simulink model "GlideslopeAndFlare"  (R2021b)
settings: Solver=VariableStepAuto  StartTime=0.0  StopTime=150  RelTol=1e-3
values from neighbouring files (symbols this model uses):
  alpha0 = trim_state_lo(8)    [Glideslope.m]
  coeff_x = x0/sqrt(x0^2+y0^2)    [Glideslope.m]
  coeff_y = y0/sqrt(x0^2+y0^2)    [Glideslope.m]
  h_flare = 19.1817    [Glideslope.m]
  max_dev_elevator = 25 - trim_control_lo(1)    [Glideslope.m]
  max_dev_thrust = 19000 - trim_thrust_lo    [Glideslope.m]
  min_dev_elevator = -25 - trim_control_lo(1)    [Glideslope.m]
  min_dev_thrust = 1000 - trim_thrust_lo    [Glideslope.m]
  tau = 1.2217    [Glideslope.m]
  theta0 = trim_state_lo(5)    [Glideslope.m]
  x0 = 3000 + 2000/(3*pi/180)    (= 41197.1863421)    [Glideslope.m]
undefined symbols (not defined in the file or in its folder): magnitude
libraries: slpidlib x2, cstblocks x1
settings Model: Creator=misha  LastModifiedBy=20181021

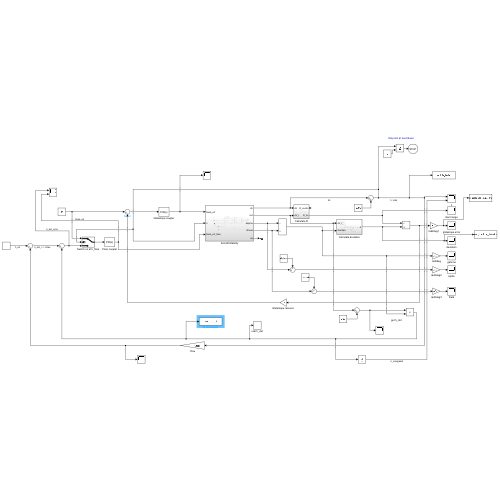
[thumbnail: Simulink's stored preview of the top-level diagram]
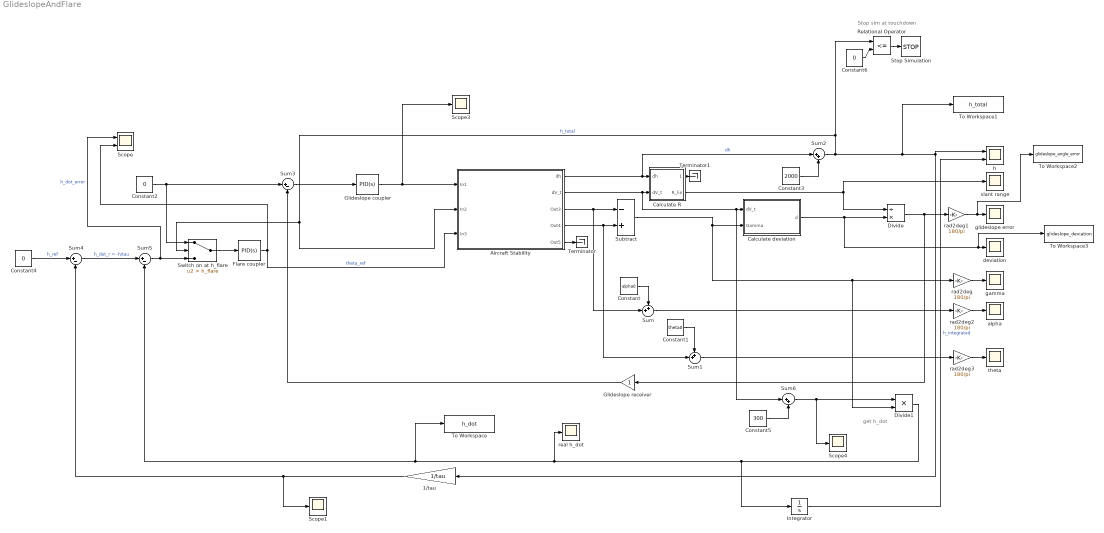
== system GlideslopeAndFlare ==
  note: Stop sim at touchdown
  note: get h_dot
  1/tau : Gain  Gain=1/tau
  Aircraft Stability : Subsystem
  Calculate R : Subsystem
  Calculate deviation : Subsystem
  Constant : Constant  Value=alpha0
  Constant1 : Constant  Value=theta0
  Constant2 : Constant  Value=0
  Constant3 : Constant  Value=2000
  Constant4 : Constant  Value=0
  Constant5 : Constant  Value=300
  Constant6 : Constant  Value=0
  Divide : Product  Inputs=/*
  Divide1 : Product  Inputs=**
  Flare coupler : slpidlib/PID Controller  Controller=PID  Form=Parallel  TimeDomain=Continuous-time  UseExternalTs=off  SampleTime=-1  IntegratorMethod=Forward Euler  FilterMethod=Forward Euler  ControllerParametersSource=internal  P=0.205  I=0.0205  D=0  UseFilter=on  N=100  TunerSelectOption=Transfer Function Based (PID Tuner App)  InitialConditionSource=internal  InitialConditionForIntegrator=0  InitialConditionForFilter=0  DifferentiatorICPrevScaledInput=0  ExternalReset=none  TrackingMode=off  Kt=1  LimitOutput=off  SatLimitsSource=internal  UpperSaturationLimit=inf  LowerSaturationLimit=-inf  LinearizeAsGain=on  AntiWindupMode=none  Kb=1  POutMin=[]  POutMax=[]  IOutMin=[]  IOutMax=[]  DOutMin=[]  DOutMax=[]  NOutMin=[]  NOutMax=[]  SumOutMin=[]  SumOutMax=[]  SaturationOutMin=[]  SaturationOutMax=[]  PParamMin=[]  PParamMax=[]  IParamMin=[]  IParamMax=[]  DParamMin=[]  DParamMax=[]  NParamMin=[]  NParamMax=[]  KbParamMin=[]  KbParamMax=[]  KtParamMin=[]  KtParamMax=[]  KbOutMin=[]  KbOutMax=[]  KtOutMin=[]  KtOutMax=[]  IntegratorOutMin=[]  IntegratorOutMax=[]  FilterOutMin=[]  FilterOutMax=[]  SumI1OutMin=[]  SumI1OutMax=[]  SumI2OutMin=[]  SumI2OutMax=[]  SumI3OutMin=[]  SumI3OutMax=[]  SumI4OutMin=[]  SumI4OutMax=[]  SumDOutMin=[]  SumDOutMax=[]  DifferentiatorOutMin=[]  DifferentiatorOutMax=[]  FilterDiffOutCoefMin=[]  FilterDiffOutCoefMax=[]  ReciprocalOutMin=[]  ReciprocalOutMax=[]  SumDenOutMin=[]  SumDenOutMax=[]  SumNumOutMin=[]  SumNumOutMax=[]  DivideOutMin=[]  DivideOutMax=[]  UdiffTsProdOutMin=[]  UdiffTsProdOutMax=[]  NTsProdOutMin=[]  NTsProdOutMax=[]  UintegralTsProdOutMin=[]  UintegralTsProdOutMax=[]  UngainTsProdOutMin=[]  UngainTsProdOutMax=[]  IntegratorContinuousStateAttributes=''  IntegratorStateMustResolveToSignalObject=off  IntegratorRTWStateStorageClass=Auto  FilterContinuousStateAttributes=''  FilterStateMustResolveToSignalObject=off  FilterRTWStateStorageClass=Auto  ParallelPVariant=InternalParameters  IdealPVariant=Disabled  IVariant=InternalParameters  DVariant=InternalParameters  IntegratorVariant=Continuous  SatVariant=Disabled  AWVariant=Passthrough  PCopyVariant=Disabled  TRVariant=Disabled  FdbkBlocksVariant=Forward  IdealPFdbkVariant=Disabled  SatFdbkVariant=Disabled  DerivativeFilterVariant=ContFilter  NVariant=InternalParameters  NCopyVariant=Disabled  FilterICVariant=InternalICsFilter  IntegratorICVariant=InternalICs  ExternalResetVariant=Disabled  TRSumVariant=Passthrough  SumFdbkVariant=Disabled  SumVariant=Sum_PID  TsampFilterVariant=InternalTs  TsampNgainVariant=Passthrough  TsampIntegralVariant=Passthrough  ExternalSaturationOutDataTypeStr=Inherit: Same as second input
  Glideslope coupler : slpidlib/PID Controller  Controller=PID  Form=Parallel  TimeDomain=Continuous-time  UseExternalTs=off  SampleTime=-1  IntegratorMethod=Forward Euler  FilterMethod=Forward Euler  ControllerParametersSource=internal  P=2000  I=200  D=0  UseFilter=on  N=100  TunerSelectOption=Transfer Function Based (PID Tuner App)  InitialConditionSource=internal  InitialConditionForIntegrator=0  InitialConditionForFilter=0  DifferentiatorICPrevScaledInput=0  ExternalReset=none  TrackingMode=off  Kt=1  LimitOutput=off  SatLimitsSource=internal  UpperSaturationLimit=inf  LowerSaturationLimit=-inf  LinearizeAsGain=on  AntiWindupMode=none  Kb=1  POutMin=[]  POutMax=[]  IOutMin=[]  IOutMax=[]  DOutMin=[]  DOutMax=[]  NOutMin=[]  NOutMax=[]  SumOutMin=[]  SumOutMax=[]  SaturationOutMin=[]  SaturationOutMax=[]  PParamMin=[]  PParamMax=[]  IParamMin=[]  IParamMax=[]  DParamMin=[]  DParamMax=[]  NParamMin=[]  NParamMax=[]  KbParamMin=[]  KbParamMax=[]  KtParamMin=[]  KtParamMax=[]  KbOutMin=[]  KbOutMax=[]  KtOutMin=[]  KtOutMax=[]  IntegratorOutMin=[]  IntegratorOutMax=[]  FilterOutMin=[]  FilterOutMax=[]  SumI1OutMin=[]  SumI1OutMax=[]  SumI2OutMin=[]  SumI2OutMax=[]  SumI3OutMin=[]  SumI3OutMax=[]  SumI4OutMin=[]  SumI4OutMax=[]  SumDOutMin=[]  SumDOutMax=[]  DifferentiatorOutMin=[]  DifferentiatorOutMax=[]  FilterDiffOutCoefMin=[]  FilterDiffOutCoefMax=[]  ReciprocalOutMin=[]  ReciprocalOutMax=[]  SumDenOutMin=[]  SumDenOutMax=[]  SumNumOutMin=[]  SumNumOutMax=[]  DivideOutMin=[]  DivideOutMax=[]  UdiffTsProdOutMin=[]  UdiffTsProdOutMax=[]  NTsProdOutMin=[]  NTsProdOutMax=[]  UintegralTsProdOutMin=[]  UintegralTsProdOutMax=[]  UngainTsProdOutMin=[]  UngainTsProdOutMax=[]  IntegratorContinuousStateAttributes=''  IntegratorStateMustResolveToSignalObject=off  IntegratorRTWStateStorageClass=Auto  FilterContinuousStateAttributes=''  FilterStateMustResolveToSignalObject=off  FilterRTWStateStorageClass=Auto  ParallelPVariant=InternalParameters  IdealPVariant=Disabled  IVariant=InternalParameters  DVariant=InternalParameters  IntegratorVariant=Continuous  SatVariant=Disabled  AWVariant=Passthrough  PCopyVariant=Disabled  TRVariant=Disabled  FdbkBlocksVariant=Forward  IdealPFdbkVariant=Disabled  SatFdbkVariant=Disabled  DerivativeFilterVariant=ContFilter  NVariant=InternalParameters  NCopyVariant=Disabled  FilterICVariant=InternalICsFilter  IntegratorICVariant=InternalICs  ExternalResetVariant=Disabled  TRSumVariant=Passthrough  SumFdbkVariant=Disabled  SumVariant=Sum_PID  TsampFilterVariant=InternalTs  TsampNgainVariant=Passthrough  TsampIntegralVariant=Passthrough  ExternalSaturationOutDataTypeStr=Inherit: Same as second input
  Glideslope receiver : Gain
  Integrator : Integrator  InitialCondition=2000
  Relational Operator : RelationalOperator  Operator=<=  OutDataTypeStr=boolean  RndMeth=Simplest
  Scope : Scope  NumInputPorts=2
  Scope1 : Scope
  Scope3 : Scope
  Scope4 : Scope
  Stop Simulation : Stop
  Subtract : Sum  Inputs=-+
  Sum : Sum  Inputs=++|
  Sum1 : Sum  Inputs=++|
  Sum2 : Sum  Inputs=|++
  Sum3 : Sum  Inputs=|+-
  Sum4 : Sum  Inputs=|+-
  Sum5 : Sum  Inputs=|+-
  Sum6 : Sum  Inputs=|++
  Switch on at h_flare : Switch  Criteria=u2 > Threshold  Threshold=h_flare
  Terminator : Terminator
  Terminator1 : Terminator
  To Workspace : ToWorkspace  VariableName=h_dot  SampleTime=-1
      settings: Save2DSignal=2-D array (concatenate along first dimension)
  To Workspace1 : ToWorkspace  VariableName=h_total  SampleTime=-1
      settings: Save2DSignal=2-D array (concatenate along first dimension)
  To Workspace2 : ToWorkspace  VariableName=glideslope_angle_error  SampleTime=-1
      settings: Save2DSignal=2-D array (concatenate along first dimension)
  To Workspace3 : ToWorkspace  VariableName=glideslope_deviation  SampleTime=-1
      settings: Save2DSignal=2-D array (concatenate along first dimension)
  alpha : Scope
  deviation : Scope
  gamma : Scope
  glideslope error : Scope
  h : Scope  NumInputPorts=2
  rad2deg{,1..3} (4 alike) : Gain  Gain=180/pi
  real h_dot : Scope
  slant range : Scope
  theta : Scope
  wires:
  Aircraft Stability/1(dh) -> Sum2/1, Calculate R/1(dh)  "dh"
  Aircraft Stability/2(dV_t) -> Sum6/1, Calculate deviation/1(dV_t), Calculate R/2(dV_t)
  Aircraft Stability/4(Out4) -> Sum1/2, Subtract/2
  Aircraft Stability/5(Out5) -> Terminator/1
  Divide/1 -> Glideslope receiver/1, rad2deg1/1
  Glideslope receiver/1 -> Sum3/2
  Constant2/1 -> Switch on at h_flare/1, Sum3/1
  Subtract/1 -> Calculate deviation/2(Gamma), rad2deg/1, Divide1/2
  Sum3/1 -> Glideslope coupler/1
  Aircraft Stability/3(Out3) -> Subtract/1, Sum/2
  Glideslope coupler/1 -> Aircraft Stability/1(In1), Scope3/1
  rad2deg/1 -> gamma/1
  rad2deg1/1 -> To Workspace2/1, glideslope error/1
  Calculate deviation/1(d) -> Divide/2, To Workspace3/1, deviation/1
  Calculate R/1(R_nonlin) -> Terminator1/1
  Calculate R/2(R_lin) -> Divide/1, slant range/1
  Constant/1 -> Sum/1
  Constant1/1 -> Sum1/1
  rad2deg2/1 -> alpha/1
  rad2deg3/1 -> theta/1
  Sum/1 -> rad2deg2/1
  Sum1/1 -> rad2deg3/1
  Constant3/1 -> Sum2/2
  Sum2/1 -> Relational Operator/1, Aircraft Stability/2(In2), Switch on at h_flare/2, To Workspace1/1, 1/tau/1, h/1  "h_total"
  Constant4/1 -> Sum4/1  "h_ref"
  Sum4/1 -> Sum5/1  "h_dot_r = -h/tau"
  Constant5/1 -> Sum6/2
  Sum6/1 -> Divide1/1, Scope4/1
  Divide1/1 -> To Workspace/1, Sum5/2, real h_dot/1, Integrator/1
  Sum5/1 -> Switch on at h_flare/3, Scope/1  "h_dot_error"
  Relational Operator/1 -> Stop Simulation/1
  Constant6/1 -> Relational Operator/2
  Flare coupler/1 -> Aircraft Stability/3(In3), Scope/2  "theta_ref"
  Switch on at h_flare/1 -> Flare coupler/1
  Integrator/1 -> h/2  "h_integrated"
  1/tau/1 -> Scope1/1, Sum4/2

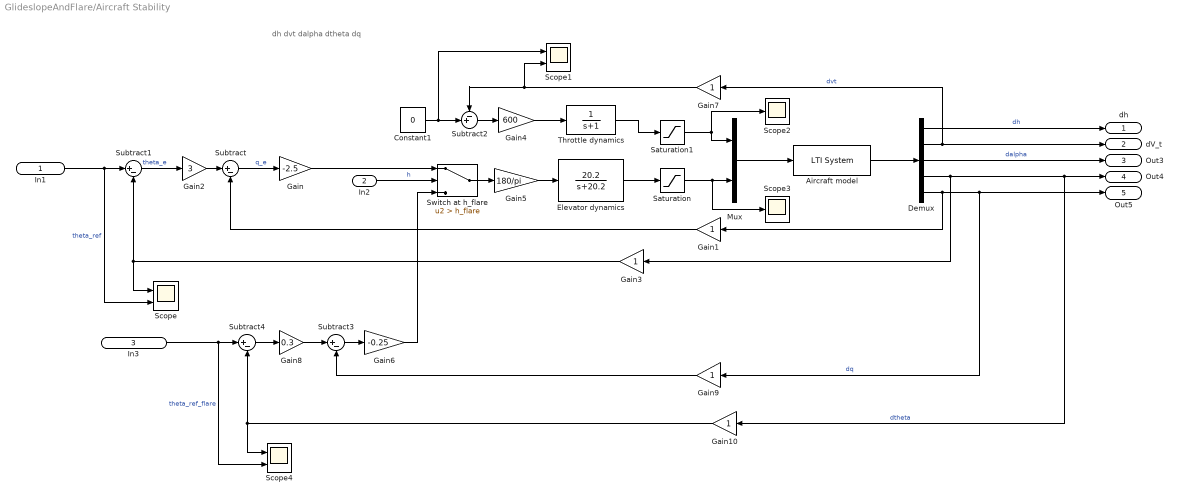
== system GlideslopeAndFlare/Aircraft Stability ==
  note: dh
      | dvt
      | dalpha
      | dtheta
      | dq
  In1 : Inport
  In2 : Inport  Port=2
  In3 : Inport  Port=3
  Aircraft model : cstblocks/LTI System  sys=sys_reduced  IC=[]
  Constant1 : Constant  Value=0
  Demux : Demux  Outputs=5
  Elevator dynamics : TransferFcn  Numerator=[20.2]  Denominator=[1 20.2]
  Gain : Gain  Gain=-2.5
  Gain{1,3,7,9..10} (5 alike) : Gain
  Gain2 : Gain  Gain=3
  Gain4 : Gain  Gain=600
  Gain5 : Gain  Gain=180/pi
  Gain6 : Gain  Gain=-0.25
  Gain8 : Gain  Gain=0.3
  Mux : Mux  Inputs=2
  Saturation : Saturate  UpperLimit=max_dev_elevator  LowerLimit=min_dev_elevator
  Saturation1 : Saturate  UpperLimit=max_dev_thrust  LowerLimit=min_dev_thrust
  Scope : Scope  NumInputPorts=2
  Scope1 : Scope  NumInputPorts=2
  Scope2 : Scope
  Scope3 : Scope
  Scope4 : Scope  NumInputPorts=2
  Subtract{,1,3..4} (4 alike) : Sum  Inputs=|+-
  Subtract2 : Sum  Inputs=-+|
  Switch at h_flare : Switch  Criteria=u2 > Threshold  Threshold=h_flare
  Throttle dynamics : TransferFcn  Denominator=[1 1]
  dh : Outport
  dV_t : Outport  Port=2
  Out3 : Outport  Port=3
  Out4 : Outport  Port=4
  Out5 : Outport  Port=5
  wires:
  Gain5/1 -> Elevator dynamics/1
  In1/1 -> Subtract1/1, Scope/2  "theta_ref"
  Demux/4 -> Gain10/1, Out4/1, Gain3/1  "dtheta"
  Gain2/1 -> Subtract/1
  Gain/1 -> Switch at h_flare/1
  Mux/1 -> Aircraft model/1
  Gain1/1 -> Subtract/2
  Gain3/1 -> Scope/1, Subtract1/2
  Saturation/1 -> Mux/2, Scope3/1
  Throttle dynamics/1 -> Saturation1/1
  Aircraft model/1 -> Demux/1
  Saturation1/1 -> Scope2/1, Mux/1
  Demux/3 -> Out3/1  "dalpha"
  Demux/2 -> dV_t/1, Gain7/1  "dvt"
  Demux/5 -> Out5/1, Gain9/1, Gain1/1  "dq"
  Subtract/1 -> Gain/1  "q_e"
  Constant1/1 -> Scope1/1, Subtract2/2
  Gain7/1 -> Scope1/2, Subtract2/1
  Demux/1 -> dh/1  "dh"
  Subtract1/1 -> Gain2/1  "theta_e"
  Elevator dynamics/1 -> Saturation/1
  Subtract2/1 -> Gain4/1
  Gain4/1 -> Throttle dynamics/1
  Switch at h_flare/1 -> Gain5/1
  In2/1 -> Switch at h_flare/2  "h"
  In3/1 -> Subtract4/1, Scope4/2  "theta_ref_flare"
  Gain8/1 -> Subtract3/1
  Subtract4/1 -> Gain8/1
  Subtract3/1 -> Gain6/1
  Gain6/1 -> Switch at h_flare/3
  Gain9/1 -> Subtract3/2
  Gain10/1 -> Subtract4/2, Scope4/1

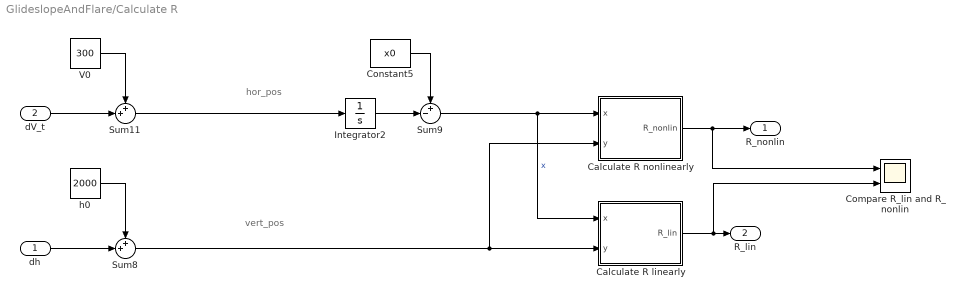
== system GlideslopeAndFlare/Calculate R ==
  note: vert_pos
  note: hor_pos
  dh : Inport
  dV_t : Inport  Port=2
  Calculate R linearly : Subsystem
  Calculate R nonlinearly : Subsystem
  Compare R_lin and R_nonlin : Scope  NumInputPorts=2
  Constant5 : Constant  Value=x0
  Integrator2 : Integrator
  Sum11 : Sum  Inputs=++|
  Sum8 : Sum  Inputs=++|
  Sum9 : Sum  Inputs=+-|
  V0 : Constant  Value=300
  h0 : Constant  Value=2000
  R_nonlin : Outport
  R_lin : Outport  Port=2
  wires:
  Sum8/1 -> Calculate R linearly/2(y), Calculate R nonlinearly/2(y)
  Sum9/1 -> Calculate R linearly/1(x), Calculate R nonlinearly/1(x)  "x"
  dh/1 -> Sum8/2
  dV_t/1 -> Sum11/2
  h0/1 -> Sum8/1
  Integrator2/1 -> Sum9/2
  Sum11/1 -> Integrator2/1
  Constant5/1 -> Sum9/1
  V0/1 -> Sum11/1
  Calculate R linearly/1(R_lin) -> Compare R_lin and R_nonlin/2, R_lin/1
  Calculate R nonlinearly/1(R_nonlin) -> Compare R_lin and R_nonlin/1, R_nonlin/1

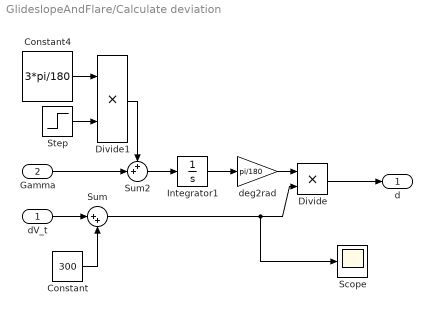
== system GlideslopeAndFlare/Calculate deviation ==
  dV_t : Inport
  Gamma : Inport  Port=2
  Constant : Constant  Value=300
  Constant4 : Constant  Value=3*pi/180
  Divide : Product  Inputs=**
  Divide1 : Product  Inputs=**
  Integrator1 : Integrator
  Scope : Scope
  Step : Step  Time=10  SampleTime=0
  Sum : Sum  Inputs=|++
  Sum2 : Sum  Inputs=++|
  deg2rad : Gain  Gain=pi/180
  d : Outport
  wires:
  Constant4/1 -> Divide1/1
  Sum2/1 -> Integrator1/1
  Gamma/1 -> Sum2/2
  Integrator1/1 -> deg2rad/1
  Step/1 -> Divide1/2
  Divide1/1 -> Sum2/1
  dV_t/1 -> Sum/1
  Constant/1 -> Sum/2
  Divide/1 -> d/1
  deg2rad/1 -> Divide/1
  Sum/1 -> Scope/1, Divide/2

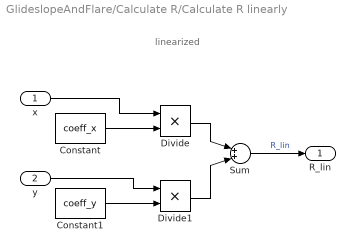
== system GlideslopeAndFlare/Calculate R/Calculate R linearly ==
  note: linearized
  x : Inport
  y : Inport  Port=2
  Constant : Constant  Value=coeff_x
  Constant1 : Constant  Value=coeff_y
  Divide : Product  Inputs=**
  Divide1 : Product  Inputs=**
  Sum : Sum  Inputs=|++|
  R_lin : Outport
  wires:
  y/1 -> Divide1/1
  Constant1/1 -> Divide1/2
  Divide/1 -> Sum/1
  Divide1/1 -> Sum/2
  Constant/1 -> Divide/2
  Sum/1 -> R_lin/1  "R_lin"
  x/1 -> Divide/1

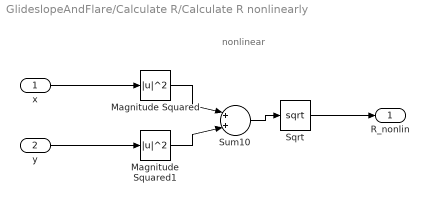
== system GlideslopeAndFlare/Calculate R/Calculate R nonlinearly ==
  note: nonlinear
  x : Inport
  y : Inport  Port=2
  Magnitude Squared : Math  Operator=magnitude^2  SaturateOnIntegerOverflow=on
  Magnitude Squared1 : Math  Operator=magnitude^2  SaturateOnIntegerOverflow=on
  Sqrt : Sqrt  SaturateOnIntegerOverflow=on
  Sum10 : Sum  Inputs=|++|
  R_nonlin : Outport
  wires:
  Magnitude Squared/1 -> Sum10/1
  Magnitude Squared1/1 -> Sum10/2
  Sum10/1 -> Sqrt/1
  Sqrt/1 -> R_nonlin/1
  x/1 -> Magnitude Squared/1
  y/1 -> Magnitude Squared1/1
